simulink model "oxidationMPC"  (R2023a)
settings: Solver=VariableStepAuto  StartTime=0.0  StopTime=Tstop  RelTol=1e-3
values from neighbouring files (symbols this model uses):
  PredictionHorizon = 10    [NonlinearAndGSMPCControlOfAnEthyleneOxidationPlant1.m]
  Ts = 5    [NonlinearAndGSMPCControlOfAnEthyleneOxidationPlant1.m]
  uLow = [0.38 0.5]    [NonlinearAndGSMPCControlOfAnEthyleneOxidationPlant1.m]
  xLow = fsolve(@(x) oxidationStateFcn(x,uLow),[1 0.3 0.03 1],options)    [NonlinearAndGSMPCControlOfAnEthyleneOxidationPlant1.m]
undefined symbols (not defined in the file or in its folder): ref
libraries: mpclib x1
settings Model: Creator=The MathWorks, Inc.  LastModifiedBy=The MathWorks, Inc.
settings SolverCC: AlgebraicLoopSolver=TrustRegion
settings DataIOCC: SaveFormat=Array  SaveOutput=off  SignalLogging=off  DSMLogging=off  SaveTime=off  ReturnWorkspaceOutputs=off
settings DebuggingCC: UnconnectedInputMsg=warning  UnconnectedOutputMsg=warning  UnconnectedLineMsg=warning  ArithmeticOperatorsInVariantConditions=warning
settings ModelReferenceCC: EnableRefExpFcnMdlSchedulingChecks=on
settings SFSimCC: SimUseLocalCustomCode=off  CustomCodeUndefinedFunction=UseInterfaceOnly
settings RTWCC: RTWUseLocalCustomCode=off
settings CodeAppCC: StateflowObjectComments=on
settings GRTTargetCC: TargetLangStandard=C89/C90 (ANSI)
settings ConfigComp: CovMetricSettings=dsw  CovSaveCumulativeToWorkspaceVar=on  CovSaveSingleToWorkspaceVar=on  CovExternalEMLEnable=off

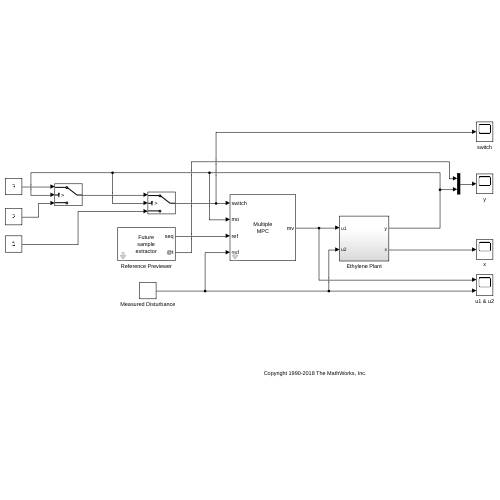
[thumbnail: Simulink's stored preview of the top-level diagram]
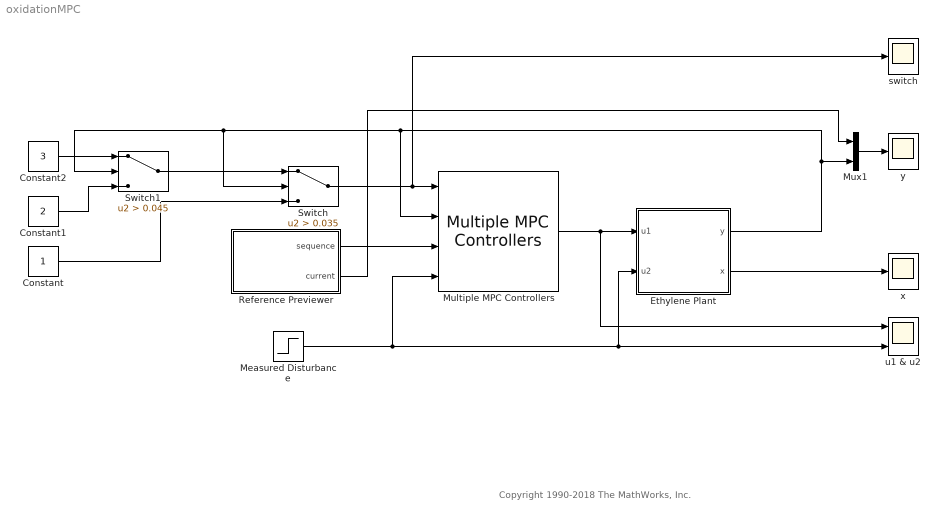
== system oxidationMPC ==
  note: Copyright 1990-2018 The MathWorks, Inc.
  Constant : Constant
  Constant1 : Constant  Value=2
  Constant2 : Constant  Value=3
  Ethylene Plant : Subsystem
  Measured Disturbance : Step  Time=200  Before=uLow(2)  After=uLow(2)+0.1  SampleTime=Ts
  Multiple MPC Controllers : mpclib/Multiple MPC Controllers  mpcobjs={'mpcobjLow' 'mpcobjMedium' 'mpcobjHigh'}  x0s={'[]' '[]' '[]'}  Nmpc=1  theMPC=1  nmv=1  nmo=1  nmd=1  nts=1  md_inport_multiple=on  mv_inport_multiple=off  uref_inport_multiple=off  return_cost_multiple=off  return_mvseq_multiple=off  return_qpstatus_multiple=off  return_xseq_multiple=off  return_state_multiple=off  return_ovseq_multiple=off  state_inport_multiple=off  umin_inport_multiple=off  umax_inport_multiple=off  ymin_inport_multiple=off  ymax_inport_multiple=off  ywt_inport_multiple=off  uwt_inport_multiple=off  duwt_inport_multiple=off  rhoeps_inport_multiple=off  BlockDataType_multiple=double  SampleTimeInherited_multiple=off
  Mux1 : Mux  Inputs=2
  Reference Previewer : Subsystem  mask{signal=ref, ts=Ts, steps=PredictionHorizon}
      mask prompts: signal "Signal name"; ts "Sampling time"; steps "Number of previewing steps"
      mask init:
      | ts = evalin('base',get_param(gcbh,'ts'));
      | signal = evalin('base',get_param(gcbh,'signal'));
      | steps = evalin('base',get_param(gcbh,'steps'));
      | data = mpc_previewer_maskinit(signal,ts);
      mask Display:
      | fprintf('Future\nsample\nextractor');
      | port_label('output', 1, 'seq')
      | port_label('output', 2, '@t')
  Switch : Switch  Criteria=u2 > Threshold  Threshold=0.035  SaturateOnIntegerOverflow=off  InputSameDT=off
  Switch1 : Switch  Criteria=u2 > Threshold  Threshold=0.045  SaturateOnIntegerOverflow=off  InputSameDT=off
  switch : Scope
  u1 & u2 : Scope  NumInputPorts=2
  x : Scope
  y : Scope
  wires:
  Mux1/1 -> y/1
  Reference Previewer/1(sequence) -> Multiple MPC Controllers/3
  Reference Previewer/2(current) -> Mux1/1
  Multiple MPC Controllers/1 -> Ethylene Plant/1(u1), u1 & u2/1
  Measured Disturbance/1 -> Ethylene Plant/2(u2), u1 & u2/2, Multiple MPC Controllers/4
  Ethylene Plant/2(x) -> x/1
  Ethylene Plant/1(y) -> Multiple MPC Controllers/2, Switch1/2, Switch/2, Mux1/2
  Switch/1 -> switch/1, Multiple MPC Controllers/1
  Constant/1 -> Switch/3
  Switch1/1 -> Switch/1
  Constant1/1 -> Switch1/3
  Constant2/1 -> Switch1/1

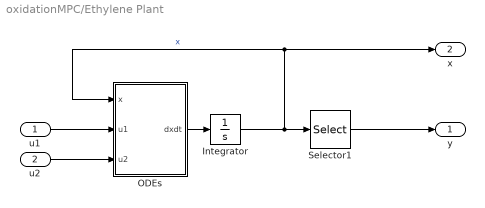
== system oxidationMPC/Ethylene Plant ==
  u1 : Inport
  u2 : Inport  Port=2
  Integrator : Integrator  InitialCondition=xLow
  ODEs : MATLAB Function  TreatAsAtomicUnit=on
  Selector1 : Selector  InputPortWidth=4  IndexOptions=Index vector (dialog)  Indices=3  OutputSizes=1
  y : Outport  VectorParamsAs1DForOutWhenUnconnected=off
  x : Outport  Port=2  VectorParamsAs1DForOutWhenUnconnected=off
  wires:
  Integrator/1 -> Selector1/1, ODEs/1(x), x/1  "x"
  ODEs/1(dxdt) -> Integrator/1
  Selector1/1 -> y/1
  u1/1 -> ODEs/2(u1)
  u2/1 -> ODEs/3(u2)

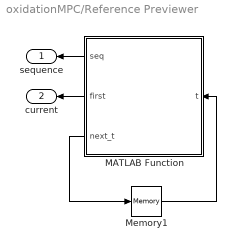
== system oxidationMPC/Reference Previewer ==
  MATLAB Function : MATLAB Function  TreatAsAtomicUnit=on
  Memory1 : Memory  InheritSampleTime=on  LinearizeAsDelay=on
  sequence : Outport  VectorParamsAs1DForOutWhenUnconnected=off
  current : Outport  Port=2  VectorParamsAs1DForOutWhenUnconnected=off
  wires:
  MATLAB Function/1(seq) -> sequence/1
  MATLAB Function/2(first) -> current/1
  Memory1/1 -> MATLAB Function/1(t)
  MATLAB Function/3(next_t) -> Memory1/1

== matlab function oxidationMPC/Reference Previewer/MATLAB Function ==
  settings: updateMethod=DISCRETE  sampleTime=ts
  data: data parameter; seq output; steps parameter; t input; first output; next_t output
function [seq,first,next_t] = fcn(data,steps,t)
%#codegen
[seq,first,next_t] = mpcblock_preview('ref',data,steps,t);

== matlab function oxidationMPC/Ethylene Plant/ODEs ==
  data: dxdt output; x input; u1 input; u2 input
function dxdt = fcn(x, u1, u2)

% Compute time derivatives and outputs for the ethylene oxide reactor

% Compute state derivatives
dxdt = oxidationStateFcn(x, [u1;u2]);
